simulink model "ILC_hardware"  (R2018a)
settings: Solver=FixedStepDiscrete  StartTime=0.0  StopTime=inf  FixedStep=0.002  RelTol=1e-3  EnableMultiTasking=on
undefined symbols (not defined in the file or in its folder): HIL, qc_get_step_size
libraries: quarc_library x13, dspswit3 x1
settings Model: SimulationMode=external  ExtModeTrigDuration=10000  Creator=Student  LastModifiedBy=Student
settings SolverCC: PositivePriorityOrder=on
settings RTWCC: SystemTargetFile=quarc_win64.tlc  TemplateMakefile=quarc_default_tmf  Description=QUARC Win64 Target
settings STFCustomTargetCC: TargetPreCompLibLocation=C:\PROGRA~3\QUARC\lib\2018a\win64\release  TargetLangStandard=C99 (ISO)  ConcurrentExecutionCompliant=on  SystemTargetFile=quarc_win64.tlc
settings GRTTargetCC: TargetPreCompLibLocation=C:\PROGRA~3\QUARC\lib\2018a\win64\release  ParMdlRefBuildCompliant=off  CompOptLevelCompliant=off  CombineOutputUpdateFcns=off  MatFileLogging=off  CPPClassGenCompliant=off  GRTInterface=on  UseToolchainInfoCompliant=off  ExtMode=on  ExtModeMexFile=quarc_comm

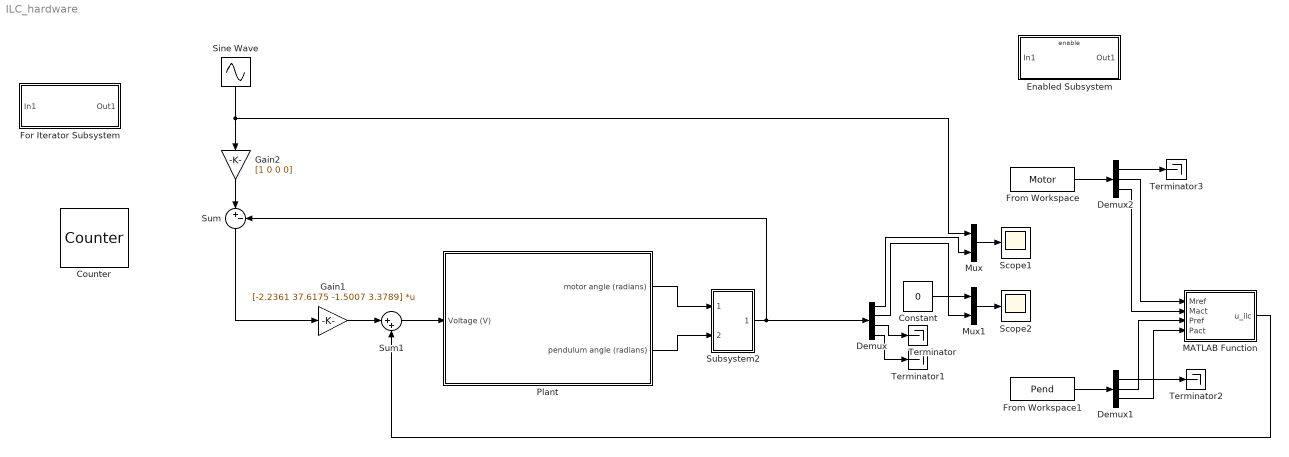
== system ILC_hardware ==
  Constant : Constant  Value=0
  Counter : dspswit3/Counter  Direction=Up  CountEvent=Rising edge  CounterSize=User defined  MaxCount=255  InitialCount=0  Output=Count and Hit  HitValue=32  ResetInput=on  SamplesPerFrame=1  Ts=1  CntDtype=double  HitDtype=Logical
  Demux : Demux
  Demux1 : Demux  Outputs=3
  Demux2 : Demux  Outputs=3
  Enabled Subsystem : Subsystem  TreatAsAtomicUnit=on
  For Iterator Subsystem : Subsystem  TreatAsAtomicUnit=on
  From Workspace : FromWorkspace  VariableName=Motor  SampleTime=0
  From Workspace1 : FromWorkspace  VariableName=Pend  SampleTime=0
  Gain1 : Gain  Gain=[-2.2361 37.6175 -1.5007 3.3789]  Multiplication=Matrix(K*u)
  Gain2 : Gain  Gain=[1 0 0 0]
  MATLAB Function : MATLAB Function  TreatAsAtomicUnit=on
  Mux : Mux  Inputs=2
  Mux1 : Mux  Inputs=2
  Plant : Subsystem
  Scope1 : Scope
  Scope2 : Scope
  Sine Wave : Sin  Frequency=2*pi  SampleTime=0
  Subsystem2 : Subsystem
  Sum : Sum  Inputs=|+-
  Sum1 : Sum  Inputs=|++
  Terminator{,1..3} (4 alike) : Terminator
  wires:
  Gain2/1 -> Sum/1
  Subsystem2/1(Out1) -> Demux/1, Sum/2
  Plant/2(pendulum angle (radians)) -> Subsystem2/2(In2)
  Sum/1 -> Gain1/1
  Plant/1(motor angle (radians)) -> Subsystem2/1(In1)
  Sine Wave/1 -> Mux/1, Gain2/1
  Mux/1 -> Scope1/1
  Sum1/1 -> Plant/1(Voltage (V))
  Gain1/1 -> Sum1/1
  Demux/1 -> Mux/2
  Mux1/1 -> Scope2/1
  Demux/2 -> Mux1/2
  Constant/1 -> Mux1/1
  Demux/3 -> Terminator/1
  Demux/4 -> Terminator1/1
  MATLAB Function/1(u_ilc) -> Sum1/2
  From Workspace1/1 -> Demux1/1
  Demux1/2 -> MATLAB Function/3(Pref)
  Demux1/3 -> MATLAB Function/4(Pact)
  Demux1/1 -> Terminator2/1
  From Workspace/1 -> Demux2/1
  Demux2/2 -> MATLAB Function/1(Mref)
  Demux2/3 -> MATLAB Function/2(Mact)
  Demux2/1 -> Terminator3/1

== system ILC_hardware/Enabled Subsystem ==
  In1 : Inport
  Enable : EnablePort
  Out1 : Outport
  wires:
  In1/1 -> Out1/1

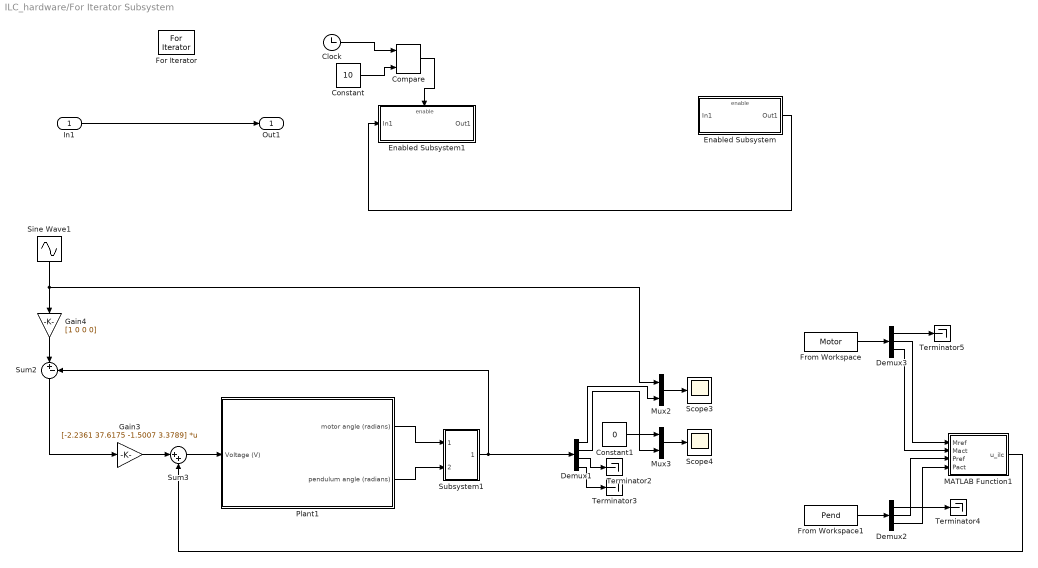
== system ILC_hardware/For Iterator Subsystem ==
  In1 : Inport
  Clock : Clock
  Compare : quarc_library/Logic Operations/Compare  operator=<  output_data_type=boolean
      settings: SourceProductName=QUARC Targets
  Constant : Constant  Value=10
  Constant1 : Constant  Value=0
  Demux1 : Demux
  Demux2 : Demux  Outputs=3
  Demux3 : Demux  Outputs=3
  Enabled Subsystem : Subsystem  TreatAsAtomicUnit=on
  Enabled Subsystem1 : Subsystem  TreatAsAtomicUnit=on
  For Iterator : ForIterator  IterationLimit=50
  From Workspace : FromWorkspace  VariableName=Motor  SampleTime=0
  From Workspace1 : FromWorkspace  VariableName=Pend  SampleTime=0
  Gain3 : Gain  Gain=[-2.2361 37.6175 -1.5007 3.3789]  Multiplication=Matrix(K*u)
  Gain4 : Gain  Gain=[1 0 0 0]
  MATLAB Function1 : MATLAB Function  TreatAsAtomicUnit=on
  Mux2 : Mux  Inputs=2
  Mux3 : Mux  Inputs=2
  Plant1 : Subsystem
  Scope3 : Scope
  Scope4 : Scope
  Sine Wave1 : Sin  Frequency=2*pi  SampleTime=0
  Subsystem1 : Subsystem
  Sum2 : Sum  Inputs=|+-
  Sum3 : Sum  Inputs=|++
  Terminator{2..5} (4 alike) : Terminator
  Out1 : Outport
  wires:
  In1/1 -> Out1/1
  Demux1/2 -> Mux3/2
  Gain3/1 -> Sum3/1
  MATLAB Function1/1(u_ilc) -> Sum3/2
  Sum3/1 -> Plant1/1(Voltage (V))
  Demux1/3 -> Terminator2/1
  Mux2/1 -> Scope3/1
  Demux1/1 -> Mux2/2
  Sine Wave1/1 -> Mux2/1, Gain4/1
  Plant1/1(motor angle (radians)) -> Subsystem1/1(In1)
  Mux3/1 -> Scope4/1
  Constant1/1 -> Mux3/1
  Plant1/2(pendulum angle (radians)) -> Subsystem1/2(In2)
  Sum2/1 -> Gain3/1
  Subsystem1/1(Out1) -> Demux1/1, Sum2/2
  Demux3/2 -> MATLAB Function1/1(Mref)
  Demux1/4 -> Terminator3/1
  Demux2/1 -> Terminator4/1
  Demux3/1 -> Terminator5/1
  From Workspace/1 -> Demux3/1
  Demux2/3 -> MATLAB Function1/4(Pact)
  Gain4/1 -> Sum2/1
  From Workspace1/1 -> Demux2/1
  Demux2/2 -> MATLAB Function1/3(Pref)
  Demux3/3 -> MATLAB Function1/2(Mact)
  Enabled Subsystem/1(Out1) -> Enabled Subsystem1/1(In1)
  Clock/1 -> Compare/1
  Constant/1 -> Compare/2
  Compare/1 -> Enabled Subsystem1/Enable

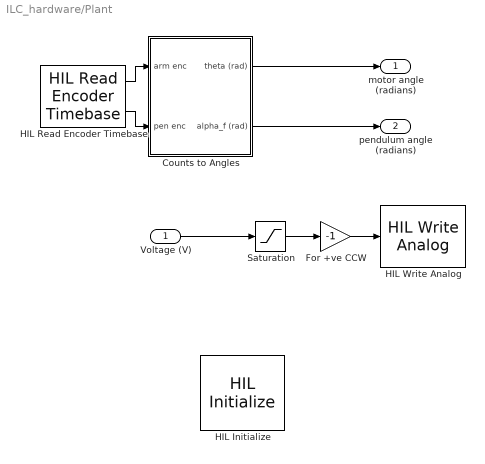
== system ILC_hardware/Plant ==
  Voltage (V) : Inport
  Counts to Angles : Subsystem
  For +ve CCW : Gain  Gain=-1
  HIL Initialize : quarc_library/Data Acquisition/Generic/Configuration/HIL Initialize  object_name=HIL-1  board_type=qube_servo2_usb  board_number=0  board_options=""  exclusive=off  active=off  hardware_clocks=[0]  clock_modes=[]  initial_clock_frequencies=[]  set_clock_params_at_start=off  set_clock_params_at_switch_in=off  set_clock_frequencies_at_start=off  set_clock_frequencies_at_switch_in=off  analog_input_channels=[0]  analog_input_configurations=[]  analog_input_maximums=3  analog_input_minimums=-3  set_analog_input_params_at_start=off  set_analog_input_params_at_switch_in=off  analog_output_channels=[0]  analog_output_maximums=15  analog_output_minimums=-15  initial_analog_outputs=[0]  final_analog_outputs=[0]  watchdog_analog_outputs=0  set_analog_output_params_at_start=off  set_analog_output_params_at_switch_in=off  set_analog_outputs_at_start=on  set_analog_outputs_at_switch_in=off  set_analog_outputs_at_terminate=on  set_analog_outputs_at_switch_out=off  set_analog_outputs_on_watchdog=on  digital_input_channels=[]  digital_output_channels=[0]  digital_output_configuration=[]  initial_digital_outputs=[1]  final_digital_outputs=[0]  watchdog_digital_outputs=[0]  set_digital_output_params_at_start=off  set_digital_output_params_at_switch_in=off  set_digital_outputs_at_start=on  set_digital_outputs_at_switch_in=off  set_digital_outputs_at_terminate=on  set_digital_outputs_at_switch_out=off  set_digital_outputs_on_watchdog=on  encoder_channels=[0:1]  quadrature=[4]  encoder_filter_frequency=[]  initial_encoder_counts=[0]  set_encoder_params_at_start=off  set_encoder_params_at_switch_in=off  set_encoder_counts_at_start=on  set_encoder_counts_at_switch_in=off  pwm_channels=[]  pwm_modes=[]  pwm_frequency=[]  pwm_configuration=[]  pwm_alignment=[]  pwm_polarity=[]  pwm_leading_deadband=[]  pwm_trailing_deadband=[]  initial_pwm_outputs=[]  final_pwm_outputs=[]  watchdog_pwm_outputs=[]  set_pwm_params_at_start=off  set_pwm_params_at_switch_in=off  set_pwm_outputs_at_start=off  set_pwm_outputs_at_switch_in=off  set_pwm_outputs_at_terminate=off  set_pwm_outputs_at_switch_out=off  set_pwm_outputs_on_watchdog=off  other_output_channels=[11000:11002]  initial_other_outputs=[0 1 0]  final_other_outputs=[1 0 0]  watchdog_other_outputs=[0 0 1]  set_other_outputs_at_start=on  set_other_outputs_at_switch_in=off  set_other_outputs_at_terminate=on  set_other_outputs_at_switch_out=off  set_other_outputs_on_watchdog=on
  HIL Read Encoder Timebase : quarc_library/Data Acquisition/Generic/Timebases/HIL Read Encoder Timebase  object_name=HIL-1  clock=0  channels=[0:1]  samples_in_buffer=max(ceil(1/qc_get_step_size), 1)  active=on  vector_output=off  data_type_mode=Inherit via back propagation  data_type=double
  HIL Write Analog : quarc_library/Data Acquisition/Generic/Immediate I//O/HIL Write Analog  object_name=HIL-1  channels=0  sample_time=-1  active=off  vector_input=off
  Saturation : Saturate  UpperLimit=10  LowerLimit=-10
  motor angle (radians) : Outport
  pendulum angle (radians) : Outport  Port=2
  wires:
  Counts to Angles/2(alpha_f (rad)) -> pendulum angle (radians)/1
  Counts to Angles/1(theta (rad)) -> motor angle (radians)/1
  For +ve CCW/1 -> HIL Write Analog/1
  Saturation/1 -> For +ve CCW/1
  Voltage (V)/1 -> Saturation/1
  HIL Read Encoder Timebase/1 -> Counts to Angles/1(arm enc)
  HIL Read Encoder Timebase/2 -> Counts to Angles/2(pen enc)

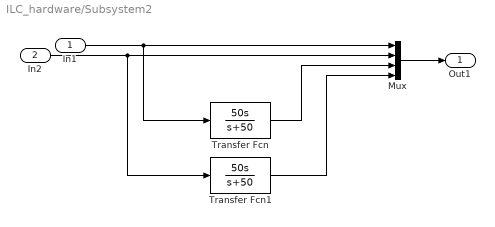
== system ILC_hardware/Subsystem2 ==
  In1 : Inport
  In2 : Inport  Port=2
  Mux : Mux
  Transfer Fcn : TransferFcn  Numerator=[50 0]  Denominator=[1 50]
  Transfer Fcn1 : TransferFcn  Numerator=[50 0]  Denominator=[1 50]
  Out1 : Outport
  wires:
  Mux/1 -> Out1/1
  Transfer Fcn/1 -> Mux/3
  In1/1 -> Transfer Fcn/1, Mux/1
  Transfer Fcn1/1 -> Mux/4
  In2/1 -> Mux/2, Transfer Fcn1/1

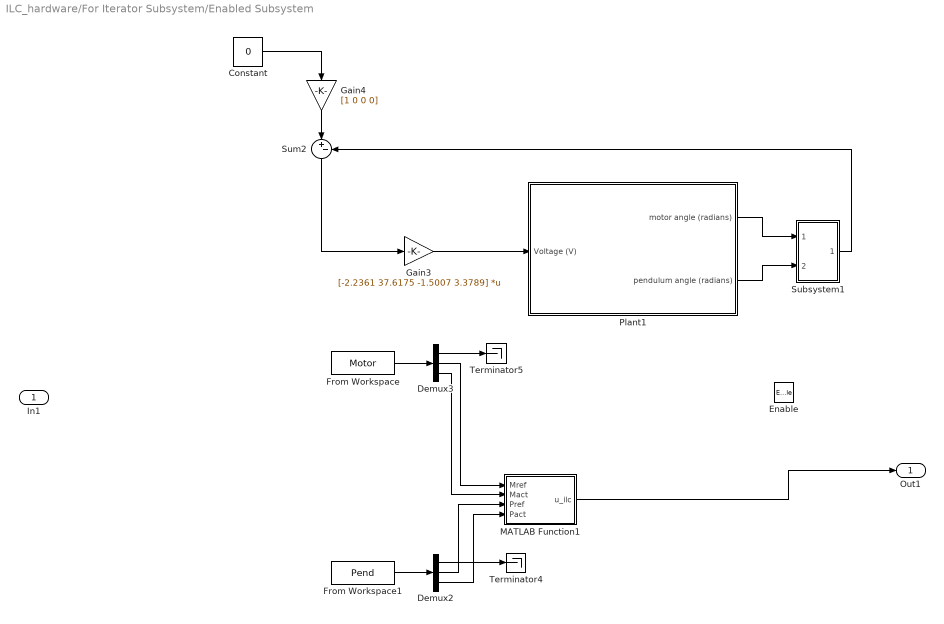
== system ILC_hardware/For Iterator Subsystem/Enabled Subsystem ==
  In1 : Inport
  Enable : EnablePort
  Constant : Constant  Value=0
  Demux2 : Demux  Outputs=3
  Demux3 : Demux  Outputs=3
  From Workspace : FromWorkspace  VariableName=Motor  SampleTime=0
  From Workspace1 : FromWorkspace  VariableName=Pend  SampleTime=0
  Gain3 : Gain  Gain=[-2.2361 37.6175 -1.5007 3.3789]  Multiplication=Matrix(K*u)
  Gain4 : Gain  Gain=[1 0 0 0]
  MATLAB Function1 : MATLAB Function  TreatAsAtomicUnit=on
  Plant1 : Subsystem
  Subsystem1 : Subsystem
  Sum2 : Sum  Inputs=|+-
  Terminator4 : Terminator
  Terminator5 : Terminator
  Out1 : Outport
  wires:
  Demux2/2 -> MATLAB Function1/3(Pref)
  Demux3/3 -> MATLAB Function1/2(Mact)
  Demux3/1 -> Terminator5/1
  Gain4/1 -> Sum2/1
  From Workspace1/1 -> Demux2/1
  From Workspace/1 -> Demux3/1
  Subsystem1/1(Out1) -> Sum2/2
  Sum2/1 -> Gain3/1
  Demux3/2 -> MATLAB Function1/1(Mref)
  Plant1/2(pendulum angle (radians)) -> Subsystem1/2(In2)
  Demux2/1 -> Terminator4/1
  Plant1/1(motor angle (radians)) -> Subsystem1/1(In1)
  Demux2/3 -> MATLAB Function1/4(Pact)
  Gain3/1 -> Plant1/1(Voltage (V))
  MATLAB Function1/1(u_ilc) -> Out1/1
  Constant/1 -> Gain4/1

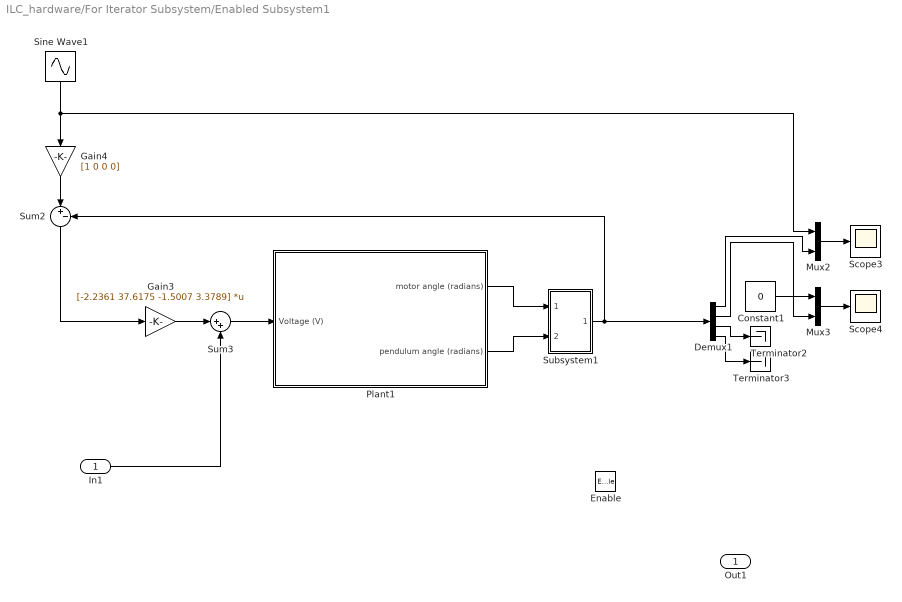
== system ILC_hardware/For Iterator Subsystem/Enabled Subsystem1 ==
  In1 : Inport
  Enable : EnablePort
  Constant1 : Constant  Value=0
  Demux1 : Demux
  Gain3 : Gain  Gain=[-2.2361 37.6175 -1.5007 3.3789]  Multiplication=Matrix(K*u)
  Gain4 : Gain  Gain=[1 0 0 0]
  Mux2 : Mux  Inputs=2
  Mux3 : Mux  Inputs=2
  Plant1 : Subsystem
  Scope3 : Scope
  Scope4 : Scope
  Sine Wave1 : Sin  Frequency=2*pi  SampleTime=0
  Subsystem1 : Subsystem
  Sum2 : Sum  Inputs=|+-
  Sum3 : Sum  Inputs=|++
  Terminator2 : Terminator
  Terminator3 : Terminator
  Out1 : Outport
  wires:
  Gain4/1 -> Sum2/1
  Subsystem1/1(Out1) -> Demux1/1, Sum2/2
  Sum2/1 -> Gain3/1
  Plant1/2(pendulum angle (radians)) -> Subsystem1/2(In2)
  Constant1/1 -> Mux3/1
  Mux3/1 -> Scope4/1
  Demux1/3 -> Terminator2/1
  Plant1/1(motor angle (radians)) -> Subsystem1/1(In1)
  Mux2/1 -> Scope3/1
  Demux1/4 -> Terminator3/1
  In1/1 -> Sum3/2
  Sine Wave1/1 -> Mux2/1, Gain4/1
  Sum3/1 -> Plant1/1(Voltage (V))
  Demux1/1 -> Mux2/2
  Demux1/2 -> Mux3/2
  Gain3/1 -> Sum3/1

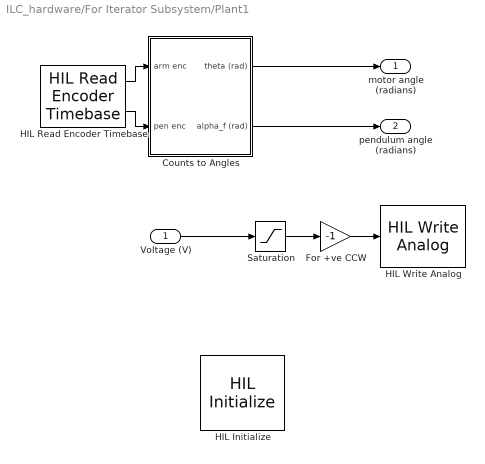
== system ILC_hardware/For Iterator Subsystem/Plant1 ==
  Voltage (V) : Inport
  Counts to Angles : Subsystem
  For +ve CCW : Gain  Gain=-1
  HIL Initialize : quarc_library/Data Acquisition/Generic/Configuration/HIL Initialize  object_name=HIL-1  board_type=qube_servo2_usb  board_number=0  board_options=""  exclusive=off  active=off  hardware_clocks=[0]  clock_modes=[]  initial_clock_frequencies=[]  set_clock_params_at_start=off  set_clock_params_at_switch_in=off  set_clock_frequencies_at_start=off  set_clock_frequencies_at_switch_in=off  analog_input_channels=[0]  analog_input_configurations=[]  analog_input_maximums=3  analog_input_minimums=-3  set_analog_input_params_at_start=off  set_analog_input_params_at_switch_in=off  analog_output_channels=[0]  analog_output_maximums=15  analog_output_minimums=-15  initial_analog_outputs=[0]  final_analog_outputs=[0]  watchdog_analog_outputs=0  set_analog_output_params_at_start=off  set_analog_output_params_at_switch_in=off  set_analog_outputs_at_start=on  set_analog_outputs_at_switch_in=off  set_analog_outputs_at_terminate=on  set_analog_outputs_at_switch_out=off  set_analog_outputs_on_watchdog=on  digital_input_channels=[]  digital_output_channels=[0]  digital_output_configuration=[]  initial_digital_outputs=[1]  final_digital_outputs=[0]  watchdog_digital_outputs=[0]  set_digital_output_params_at_start=off  set_digital_output_params_at_switch_in=off  set_digital_outputs_at_start=on  set_digital_outputs_at_switch_in=off  set_digital_outputs_at_terminate=on  set_digital_outputs_at_switch_out=off  set_digital_outputs_on_watchdog=on  encoder_channels=[0:1]  quadrature=[4]  encoder_filter_frequency=[]  initial_encoder_counts=[0]  set_encoder_params_at_start=off  set_encoder_params_at_switch_in=off  set_encoder_counts_at_start=on  set_encoder_counts_at_switch_in=off  pwm_channels=[]  pwm_modes=[]  pwm_frequency=[]  pwm_configuration=[]  pwm_alignment=[]  pwm_polarity=[]  pwm_leading_deadband=[]  pwm_trailing_deadband=[]  initial_pwm_outputs=[]  final_pwm_outputs=[]  watchdog_pwm_outputs=[]  set_pwm_params_at_start=off  set_pwm_params_at_switch_in=off  set_pwm_outputs_at_start=off  set_pwm_outputs_at_switch_in=off  set_pwm_outputs_at_terminate=off  set_pwm_outputs_at_switch_out=off  set_pwm_outputs_on_watchdog=off  other_output_channels=[11000:11002]  initial_other_outputs=[0 1 0]  final_other_outputs=[1 0 0]  watchdog_other_outputs=[0 0 1]  set_other_outputs_at_start=on  set_other_outputs_at_switch_in=off  set_other_outputs_at_terminate=on  set_other_outputs_at_switch_out=off  set_other_outputs_on_watchdog=on
  HIL Read Encoder Timebase : quarc_library/Data Acquisition/Generic/Timebases/HIL Read Encoder Timebase  object_name=HIL-1  clock=0  channels=[0:1]  samples_in_buffer=max(ceil(1/qc_get_step_size), 1)  active=on  vector_output=off  data_type_mode=Inherit via back propagation  data_type=double
  HIL Write Analog : quarc_library/Data Acquisition/Generic/Immediate I//O/HIL Write Analog  object_name=HIL-1  channels=0  sample_time=-1  active=off  vector_input=off
  Saturation : Saturate  UpperLimit=10  LowerLimit=-10
  motor angle (radians) : Outport
  pendulum angle (radians) : Outport  Port=2
  wires:
  Counts to Angles/2(alpha_f (rad)) -> pendulum angle (radians)/1
  Counts to Angles/1(theta (rad)) -> motor angle (radians)/1
  For +ve CCW/1 -> HIL Write Analog/1
  Saturation/1 -> For +ve CCW/1
  Voltage (V)/1 -> Saturation/1
  HIL Read Encoder Timebase/1 -> Counts to Angles/1(arm enc)
  HIL Read Encoder Timebase/2 -> Counts to Angles/2(pen enc)

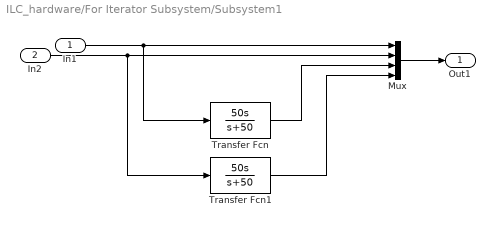
== system ILC_hardware/For Iterator Subsystem/Subsystem1 ==
  In1 : Inport
  In2 : Inport  Port=2
  Mux : Mux
  Transfer Fcn : TransferFcn  Numerator=[50 0]  Denominator=[1 50]
  Transfer Fcn1 : TransferFcn  Numerator=[50 0]  Denominator=[1 50]
  Out1 : Outport
  wires:
  Mux/1 -> Out1/1
  Transfer Fcn/1 -> Mux/3
  In1/1 -> Transfer Fcn/1, Mux/1
  Transfer Fcn1/1 -> Mux/4
  In2/1 -> Mux/2, Transfer Fcn1/1

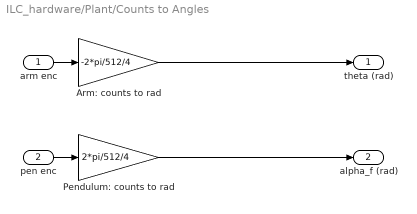
== system ILC_hardware/Plant/Counts to Angles ==
  arm enc : Inport
  pen enc : Inport  Port=2
  Arm: counts to rad : Gain  Gain=-2*pi/512/4
  Pendulum: counts to rad : Gain  Gain=2*pi/512/4
  theta (rad) : Outport
  alpha_f (rad) : Outport  Port=2
  wires:
  Arm: counts to rad/1 -> theta (rad)/1
  Pendulum: counts to rad/1 -> alpha_f (rad)/1
  arm enc/1 -> Arm: counts to rad/1
  pen enc/1 -> Pendulum: counts to rad/1

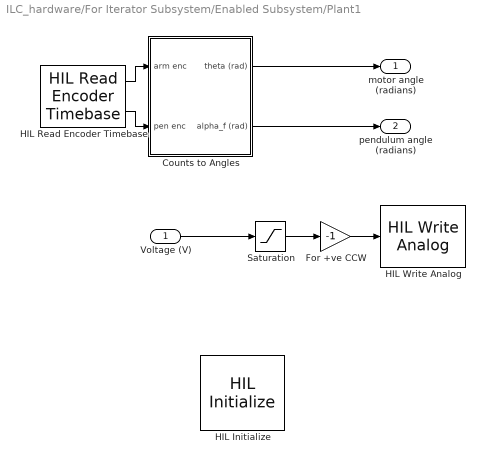
== system ILC_hardware/For Iterator Subsystem/Enabled Subsystem/Plant1 ==
  Voltage (V) : Inport
  Counts to Angles : Subsystem
  For +ve CCW : Gain  Gain=-1
  HIL Initialize : quarc_library/Data Acquisition/Generic/Configuration/HIL Initialize  object_name=HIL-1  board_type=qube_servo2_usb  board_number=0  board_options=""  exclusive=off  active=off  hardware_clocks=[0]  clock_modes=[]  initial_clock_frequencies=[]  set_clock_params_at_start=off  set_clock_params_at_switch_in=off  set_clock_frequencies_at_start=off  set_clock_frequencies_at_switch_in=off  analog_input_channels=[0]  analog_input_configurations=[]  analog_input_maximums=3  analog_input_minimums=-3  set_analog_input_params_at_start=off  set_analog_input_params_at_switch_in=off  analog_output_channels=[0]  analog_output_maximums=15  analog_output_minimums=-15  initial_analog_outputs=[0]  final_analog_outputs=[0]  watchdog_analog_outputs=0  set_analog_output_params_at_start=off  set_analog_output_params_at_switch_in=off  set_analog_outputs_at_start=on  set_analog_outputs_at_switch_in=off  set_analog_outputs_at_terminate=on  set_analog_outputs_at_switch_out=off  set_analog_outputs_on_watchdog=on  digital_input_channels=[]  digital_output_channels=[0]  digital_output_configuration=[]  initial_digital_outputs=[1]  final_digital_outputs=[0]  watchdog_digital_outputs=[0]  set_digital_output_params_at_start=off  set_digital_output_params_at_switch_in=off  set_digital_outputs_at_start=on  set_digital_outputs_at_switch_in=off  set_digital_outputs_at_terminate=on  set_digital_outputs_at_switch_out=off  set_digital_outputs_on_watchdog=on  encoder_channels=[0:1]  quadrature=[4]  encoder_filter_frequency=[]  initial_encoder_counts=[0]  set_encoder_params_at_start=off  set_encoder_params_at_switch_in=off  set_encoder_counts_at_start=on  set_encoder_counts_at_switch_in=off  pwm_channels=[]  pwm_modes=[]  pwm_frequency=[]  pwm_configuration=[]  pwm_alignment=[]  pwm_polarity=[]  pwm_leading_deadband=[]  pwm_trailing_deadband=[]  initial_pwm_outputs=[]  final_pwm_outputs=[]  watchdog_pwm_outputs=[]  set_pwm_params_at_start=off  set_pwm_params_at_switch_in=off  set_pwm_outputs_at_start=off  set_pwm_outputs_at_switch_in=off  set_pwm_outputs_at_terminate=off  set_pwm_outputs_at_switch_out=off  set_pwm_outputs_on_watchdog=off  other_output_channels=[11000:11002]  initial_other_outputs=[0 1 0]  final_other_outputs=[1 0 0]  watchdog_other_outputs=[0 0 1]  set_other_outputs_at_start=on  set_other_outputs_at_switch_in=off  set_other_outputs_at_terminate=on  set_other_outputs_at_switch_out=off  set_other_outputs_on_watchdog=on
  HIL Read Encoder Timebase : quarc_library/Data Acquisition/Generic/Timebases/HIL Read Encoder Timebase  object_name=HIL-1  clock=0  channels=[0:1]  samples_in_buffer=max(ceil(1/qc_get_step_size), 1)  active=on  vector_output=off  data_type_mode=Inherit via back propagation  data_type=double
  HIL Write Analog : quarc_library/Data Acquisition/Generic/Immediate I//O/HIL Write Analog  object_name=HIL-1  channels=0  sample_time=-1  active=off  vector_input=off
  Saturation : Saturate  UpperLimit=10  LowerLimit=-10
  motor angle (radians) : Outport
  pendulum angle (radians) : Outport  Port=2
  wires:
  Counts to Angles/2(alpha_f (rad)) -> pendulum angle (radians)/1
  Counts to Angles/1(theta (rad)) -> motor angle (radians)/1
  For +ve CCW/1 -> HIL Write Analog/1
  Saturation/1 -> For +ve CCW/1
  Voltage (V)/1 -> Saturation/1
  HIL Read Encoder Timebase/1 -> Counts to Angles/1(arm enc)
  HIL Read Encoder Timebase/2 -> Counts to Angles/2(pen enc)

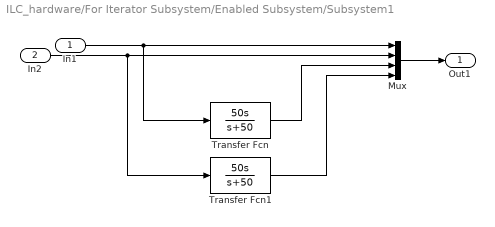
== system ILC_hardware/For Iterator Subsystem/Enabled Subsystem/Subsystem1 ==
  In1 : Inport
  In2 : Inport  Port=2
  Mux : Mux
  Transfer Fcn : TransferFcn  Numerator=[50 0]  Denominator=[1 50]
  Transfer Fcn1 : TransferFcn  Numerator=[50 0]  Denominator=[1 50]
  Out1 : Outport
  wires:
  Mux/1 -> Out1/1
  Transfer Fcn/1 -> Mux/3
  In1/1 -> Transfer Fcn/1, Mux/1
  Transfer Fcn1/1 -> Mux/4
  In2/1 -> Mux/2, Transfer Fcn1/1

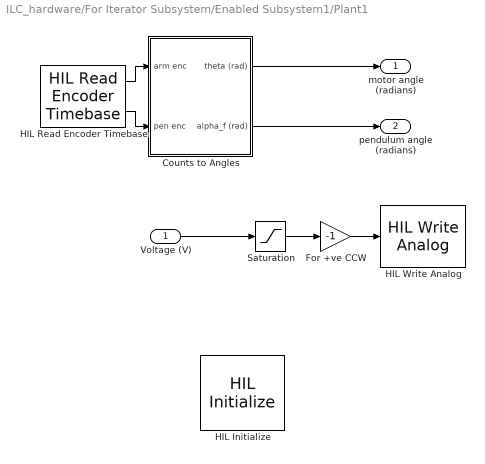
== system ILC_hardware/For Iterator Subsystem/Enabled Subsystem1/Plant1 ==
  Voltage (V) : Inport
  Counts to Angles : Subsystem
  For +ve CCW : Gain  Gain=-1
  HIL Initialize : quarc_library/Data Acquisition/Generic/Configuration/HIL Initialize  object_name=HIL-1  board_type=qube_servo2_usb  board_number=0  board_options=""  exclusive=off  active=off  hardware_clocks=[0]  clock_modes=[]  initial_clock_frequencies=[]  set_clock_params_at_start=off  set_clock_params_at_switch_in=off  set_clock_frequencies_at_start=off  set_clock_frequencies_at_switch_in=off  analog_input_channels=[0]  analog_input_configurations=[]  analog_input_maximums=3  analog_input_minimums=-3  set_analog_input_params_at_start=off  set_analog_input_params_at_switch_in=off  analog_output_channels=[0]  analog_output_maximums=15  analog_output_minimums=-15  initial_analog_outputs=[0]  final_analog_outputs=[0]  watchdog_analog_outputs=0  set_analog_output_params_at_start=off  set_analog_output_params_at_switch_in=off  set_analog_outputs_at_start=on  set_analog_outputs_at_switch_in=off  set_analog_outputs_at_terminate=on  set_analog_outputs_at_switch_out=off  set_analog_outputs_on_watchdog=on  digital_input_channels=[]  digital_output_channels=[0]  digital_output_configuration=[]  initial_digital_outputs=[1]  final_digital_outputs=[0]  watchdog_digital_outputs=[0]  set_digital_output_params_at_start=off  set_digital_output_params_at_switch_in=off  set_digital_outputs_at_start=on  set_digital_outputs_at_switch_in=off  set_digital_outputs_at_terminate=on  set_digital_outputs_at_switch_out=off  set_digital_outputs_on_watchdog=on  encoder_channels=[0:1]  quadrature=[4]  encoder_filter_frequency=[]  initial_encoder_counts=[0]  set_encoder_params_at_start=off  set_encoder_params_at_switch_in=off  set_encoder_counts_at_start=on  set_encoder_counts_at_switch_in=off  pwm_channels=[]  pwm_modes=[]  pwm_frequency=[]  pwm_configuration=[]  pwm_alignment=[]  pwm_polarity=[]  pwm_leading_deadband=[]  pwm_trailing_deadband=[]  initial_pwm_outputs=[]  final_pwm_outputs=[]  watchdog_pwm_outputs=[]  set_pwm_params_at_start=off  set_pwm_params_at_switch_in=off  set_pwm_outputs_at_start=off  set_pwm_outputs_at_switch_in=off  set_pwm_outputs_at_terminate=off  set_pwm_outputs_at_switch_out=off  set_pwm_outputs_on_watchdog=off  other_output_channels=[11000:11002]  initial_other_outputs=[0 1 0]  final_other_outputs=[1 0 0]  watchdog_other_outputs=[0 0 1]  set_other_outputs_at_start=on  set_other_outputs_at_switch_in=off  set_other_outputs_at_terminate=on  set_other_outputs_at_switch_out=off  set_other_outputs_on_watchdog=on
  HIL Read Encoder Timebase : quarc_library/Data Acquisition/Generic/Timebases/HIL Read Encoder Timebase  object_name=HIL-1  clock=0  channels=[0:1]  samples_in_buffer=max(ceil(1/qc_get_step_size), 1)  active=on  vector_output=off  data_type_mode=Inherit via back propagation  data_type=double
  HIL Write Analog : quarc_library/Data Acquisition/Generic/Immediate I//O/HIL Write Analog  object_name=HIL-1  channels=0  sample_time=-1  active=off  vector_input=off
  Saturation : Saturate  UpperLimit=10  LowerLimit=-10
  motor angle (radians) : Outport
  pendulum angle (radians) : Outport  Port=2
  wires:
  Counts to Angles/2(alpha_f (rad)) -> pendulum angle (radians)/1
  Counts to Angles/1(theta (rad)) -> motor angle (radians)/1
  For +ve CCW/1 -> HIL Write Analog/1
  Saturation/1 -> For +ve CCW/1
  Voltage (V)/1 -> Saturation/1
  HIL Read Encoder Timebase/1 -> Counts to Angles/1(arm enc)
  HIL Read Encoder Timebase/2 -> Counts to Angles/2(pen enc)

== system ILC_hardware/For Iterator Subsystem/Enabled Subsystem1/Subsystem1 ==
  In1 : Inport
  In2 : Inport  Port=2
  Mux : Mux
  Transfer Fcn : TransferFcn  Numerator=[50 0]  Denominator=[1 50]
  Transfer Fcn1 : TransferFcn  Numerator=[50 0]  Denominator=[1 50]
  Out1 : Outport
  wires:
  Mux/1 -> Out1/1
  Transfer Fcn/1 -> Mux/3
  In1/1 -> Transfer Fcn/1, Mux/1
  Transfer Fcn1/1 -> Mux/4
  In2/1 -> Mux/2, Transfer Fcn1/1

== system ILC_hardware/For Iterator Subsystem/Plant1/Counts to Angles ==
  arm enc : Inport
  pen enc : Inport  Port=2
  Arm: counts to rad : Gain  Gain=-2*pi/512/4
  Pendulum: counts to rad : Gain  Gain=2*pi/512/4
  theta (rad) : Outport
  alpha_f (rad) : Outport  Port=2
  wires:
  Arm: counts to rad/1 -> theta (rad)/1
  Pendulum: counts to rad/1 -> alpha_f (rad)/1
  arm enc/1 -> Arm: counts to rad/1
  pen enc/1 -> Pendulum: counts to rad/1

== system ILC_hardware/For Iterator Subsystem/Enabled Subsystem/Plant1/Counts to Angles ==
  arm enc : Inport
  pen enc : Inport  Port=2
  Arm: counts to rad : Gain  Gain=-2*pi/512/4
  Pendulum: counts to rad : Gain  Gain=2*pi/512/4
  theta (rad) : Outport
  alpha_f (rad) : Outport  Port=2
  wires:
  Arm: counts to rad/1 -> theta (rad)/1
  Pendulum: counts to rad/1 -> alpha_f (rad)/1
  arm enc/1 -> Arm: counts to rad/1
  pen enc/1 -> Pendulum: counts to rad/1

== system ILC_hardware/For Iterator Subsystem/Enabled Subsystem1/Plant1/Counts to Angles ==
  arm enc : Inport
  pen enc : Inport  Port=2
  Arm: counts to rad : Gain  Gain=-2*pi/512/4
  Pendulum: counts to rad : Gain  Gain=2*pi/512/4
  theta (rad) : Outport
  alpha_f (rad) : Outport  Port=2
  wires:
  Arm: counts to rad/1 -> theta (rad)/1
  Pendulum: counts to rad/1 -> alpha_f (rad)/1
  arm enc/1 -> Arm: counts to rad/1
  pen enc/1 -> Pendulum: counts to rad/1

== matlab function ILC_hardware/For Iterator Subsystem/Enabled Subsystem/MATLAB Function1 ==
  data: Mref input; u_ilc output; Mact input; Pref input; Pact input
function u_ilc = fcn(Mref, Mact, Pref, Pact)

TotalTime = 10.0 %secs
T = 0.002; %secs
time = 0:T:TotalTime;
tLen = length(time);
u_ilc = [time zeros(tLen,1)];
L = [K(1) K(2)];

for ii = 1:tLen-1
    u_ilc(ii,2) = u_ilc(ii,2) + alpha*L*[Mref(ii+1)-Mact(ii+1); Pref(ii+1)-Pact(ii+1)];
end

== matlab function ILC_hardware/MATLAB Function ==
  data: Mref input; u_ilc output; Mact input; Pref input; Pact input
function u_ilc = fcn(Mref, Mact, Pref, Pact)

TotalTime = 10.0 %secs
T = 0.002; %secs
time = 0:T:TotalTime;
tLen = length(time);
u_ilc = [time zeros(tLen,1)];
L = [K(1) K(2)];

for ii = 1:tLen-1
    u_ilc(ii,2) = u_ilc(ii,2) + alpha*L*[Mref(ii+1)-Mact(ii+1); Pref(ii+1)-Pact(ii+1)];
end
clear Motor Pend;

== matlab function ILC_hardware/For Iterator Subsystem/MATLAB Function1 ==
  data: Mref input; u_ilc output; Mact input; Pref input; Pact input
function u_ilc = fcn(Mref, Mact, Pref, Pact)

TotalTime = 10.0 %secs
T = 0.002; %secs
time = 0:T:TotalTime;
tLen = length(time);
u_ilc = [time zeros(tLen,1)];
L = [K(1) K(2)];

for ii = 1:tLen-1
    u_ilc(ii,2) = u_ilc(ii,2) + alpha*L*[Mref(ii+1)-Mact(ii+1); Pref(ii+1)-Pact(ii+1)];
end
